simulink model "skipper_lqi_for_export"  (R2025b)
settings: Solver=FixedStepDiscrete  StartTime=0.0  StopTime=100  RelTol=1e-3
values from neighbouring files (symbols this model uses):
  A = [ ... (first row only)    [lqrMatrices.m]    (also in state_space.m)
  B = [ ... (first row only)    [lqrMatrices.m]    (also in state_space.m)
  C = diag(ones(1, 12))    [lqrMatrices.m]    (also in state_space.m = eye(12))
  D = zeros(size(B))    [lqrMatrices.m]    (also in state_space.m)
  d = [-rho 0 0]'    [derive_eom.m]    (also in lqrMatrices.m = [; state_space.m = [)
  K1 = Ki(:, 1:12)    [state_space.m]
  K2 = Ki(:, 13:end)    [state_space.m]
  qq = diag([1 1 1 0.001 0.001 0.001 1 1 1 0.001 0.001 0.001])    [state_space.m]
  Uff = -pinv(B)*d    [state_space.m]
undefined symbols (not defined in the file or in its folder): DiscIntNeverNeededParam, Discrete, Time
libraries: ctrlSharedLib x1
settings Model: Creator=nehir  LastModifiedBy=turbohirbo
settings OptimizationCC: DefaultParameterBehavior=Inlined  UseDivisionForNetSlopeComputation=on  GainParamInheritBuiltInType=on  UseFloatMulNetSlope=on  InlineInvariantSignals=on  ZeroExternalMemoryAtStartup=off  ZeroInternalMemoryAtStartup=off  EfficientFloat2IntCast=on  LifeSpan=1  OptimizeDataStoreBuffers=off  BusAssignmentInplaceUpdate=off
settings DebuggingCC: SFUnexpectedBacktrackingDiag=warning  SFNoUnconditionalDefaultTransitionDiag=warning
settings HardwareCC: ProdBitPerPointer=32.0  ProdBitPerSizeT=32.0  ProdBitPerPtrDiffT=32.0  ProdLargestAtomicInteger=Long  ProdLargestAtomicFloat=Double  ProdWordSize=32.0  ProdHWDeviceType=ARM Compatible->ARM Cortex-M
settings SFSimCC: MATLABDynamicMemAlloc=off
settings RTWCC: GenCodeOnly=on  GenerateReport=on  Toolchain=CMake  LaunchReport=on  TargetLang=C++
settings CodeAppCC: ForceParamTrailComments=on  EnableCustomComments=on
settings GRTTargetCC: MultiInstanceErrorCode=Warning  TargetLangStandard=C++17 (ISO)  CombineSignalStateStructs=on  MatFileLogging=off  CodeInterfacePackaging=C++ class  SupportVariableSizeSignals=on
settings SimscapeCC: SimscapeLogDecimation=1  SimscapeLogDataHistory=5000

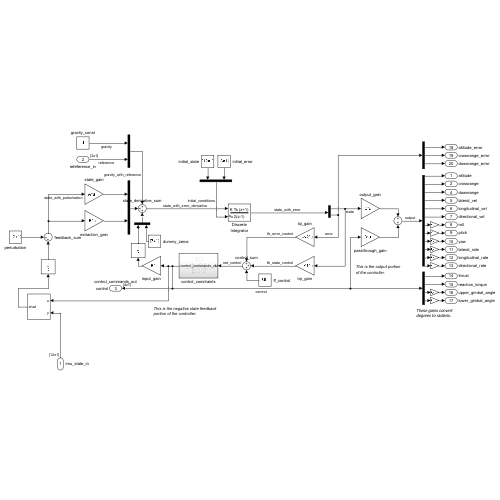
[thumbnail: Simulink's stored preview of the top-level diagram]
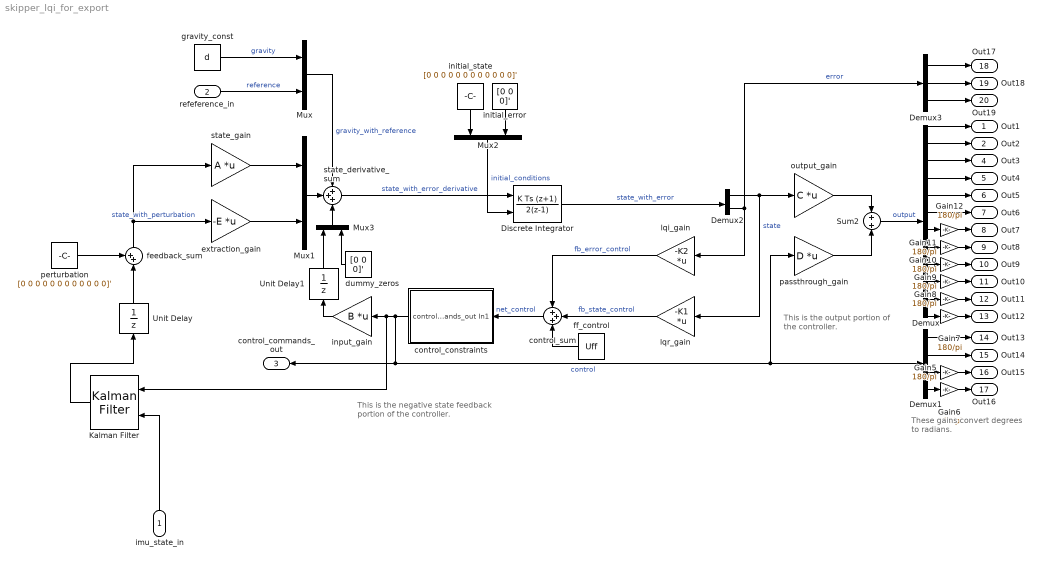
== system skipper_lqi_for_export ==
  note: This is the output portion
      | of the controller.
  note: This is the negative state feedback
      | portion of the controller.
  note: These gains convert
      | degrees to radians.
  imu_state_in : Inport  PortDimensions=[12 1]
  refeference_in : Inport  Port=2  PortDimensions=[3 1]
  Demux : Demux  Outputs=12
  Demux1 : Demux
  Demux2 : Demux  Outputs=[12 3]
  Demux3 : Demux  Outputs=3
  Discrete Integrator : DiscreteIntegrator  IntegratorMethod=Integration: Trapezoidal  InitialConditionSource=external  SampleTime=0.05  ICPrevOutput=DiscIntNeverNeededParam  ICPrevScaledInput=DiscIntNeverNeededParam
  Gain{5..12} (8 alike) : Gain  Gain=180/pi
  Kalman Filter : ctrlSharedLib/Kalman Filter  TimeDomain=Discrete-Time  UseCurrentEstimator=on  ModelSource=Individual A, B, C, D matrices  ModelSourceVariable=ss(0.95,1,1,0,1)  A=A  B=B  C=C  D=D  NumberOfStates=1  NumberOfInputs=1  NumberOfOutputs=1  InitialEstimateSource=Dialog  X0=0  P0=10  UseK=off  UseGH=off  NumberOfProcessNoiseInputs=1  G=1  TimeInvariantG=on  H=0  TimeInvariantH=on  Q=qq ./ 1  TimeInvariantQ=on  R=.01  TimeInvariantR=on  N=0  TimeInvariantN=on  AddInputPort=on  AddEnablePort=off  OutputEstimatedY=off  OutputP=off  Ts=-1
  Mux{,1..3} (4 alike) : Mux  Inputs=2
  Sum2 : Sum  Inputs=+|+
  Unit Delay : UnitDelay  SampleTime=0.05  HasFrameUpgradeWarning=on
  Unit Delay1 : UnitDelay  SampleTime=0.05  HasFrameUpgradeWarning=on
  control_constraints : Subsystem
  control_sum : Sum  Inputs=+++
  dummy_zeros : Constant  Value=[0 0 0]'  OutDataTypeStr=Inherit: Inherit via back propagation
  extraction_gain : Gain  Gain=-E  Multiplication=Matrix(K*u)
  feedback_sum : Sum  Inputs=++|
  ff_control : Constant  Value=Uff
  gravity_const : Constant  Value=d  OutDataTypeStr=double
  initial_error : Constant  Value=[0 0 0]'
  initial_state : Constant  Value=[0 0 0 0 0 0 0 0 0 0 0 0]'
  input_gain : Gain  Gain=B  Multiplication=Matrix(K*u)
  lqi_gain : Gain  Gain=-K2  Multiplication=Matrix(K*u)
  lqr_gain : Gain  Gain=-K1  Multiplication=Matrix(K*u)
  output_gain : Gain  Gain=C  Multiplication=Matrix(K*u)
  passthrough_gain : Gain  Gain=D  Multiplication=Matrix(K*u)
  perturbation : Constant  Value=[0 0 0 0 0 0 0 0 0 0 0 0]'
  state_derivative_sum : Sum  Inputs=+++
  state_gain : Gain  Gain=A  Multiplication=Matrix(K*u)
  Out1 : Outport  SignalName=altitude  Unit=ft
  Out2 : Outport  Port=2  SignalName=crossrange  Unit=ft
  control_commands_out : Outport  Port=3  SignalName=control  PortDimensions=[4 1]
  Out3 : Outport  Port=4  SignalName=downrange  Unit=ft
  Out4 : Outport  Port=5  SignalName=lateral_vel  Unit=ft/s
  Out5 : Outport  Port=6  SignalName=longitudinal_vel  Unit=ft/s
  Out6 : Outport  Port=7  SignalName=directional_vel  Unit=ft/s
  Out7 : Outport  Port=8  SignalName=roll  Unit=deg
  Out8 : Outport  Port=9  SignalName=pitch  Unit=deg
  Out9 : Outport  Port=10  SignalName=yaw  Unit=deg
  Out10 : Outport  Port=11  SignalName=lateral_rate  Unit=deg/s
  Out11 : Outport  Port=12  SignalName=longitudinal_rate  Unit=deg/s
  Out12 : Outport  Port=13  SignalName=directional_rate  Unit=deg/s
  Out13 : Outport  Port=14  SignalName=thrust  Unit=lbf
  Out14 : Outport  Port=15  SignalName=reaction_torque  Unit=lbf*ft
  Out15 : Outport  Port=16  SignalName=upper_gimbal_angle  Unit=deg
  Out16 : Outport  Port=17  SignalName=lower_gimbal_angle  Unit=deg
  Out17 : Outport  Port=18  SignalName=altitude_error  Unit=ft*s
  Out18 : Outport  Port=19  SignalName=crossrange_error  Unit=ft*s
  Out19 : Outport  Port=20  SignalName=downrange_error  Unit=ft*s
  wires:
  state_gain/1 -> Mux1/1
  input_gain/1 -> Unit Delay1/1
  state_derivative_sum/1 -> Discrete Integrator/1  "state_with_error_derivative"
  Discrete Integrator/1 -> Demux2/1  "state_with_error"
  output_gain/1 -> Sum2/1
  passthrough_gain/1 -> Sum2/2
  ff_control/1 -> control_sum/3
  lqr_gain/1 -> control_sum/2  "fb_state_control"
  control_sum/1 -> control_constraints/1(In1)  "net_control"
  initial_state/1 -> Mux2/1
  Sum2/1 -> Demux/1  "output"
  Demux/1 -> Out1/1
  Demux/2 -> Out2/1
  Demux/3 -> Out3/1
  Demux/4 -> Out4/1
  Demux/5 -> Out5/1
  Demux/6 -> Out6/1
  Demux1/1 -> Out13/1
  Demux1/2 -> Out14/1
  Demux1/3 -> Gain5/1
  Gain5/1 -> Out15/1
  Gain6/1 -> Out16/1
  Demux1/4 -> Gain6/1
  Demux/12 -> Gain7/1
  Gain7/1 -> Out12/1
  Demux/11 -> Gain8/1
  Demux/9 -> Gain10/1
  Demux/7 -> Gain12/1
  Demux/8 -> Gain11/1
  Demux/10 -> Gain9/1
  Gain12/1 -> Out7/1
  Gain11/1 -> Out8/1
  Gain10/1 -> Out9/1
  Gain9/1 -> Out10/1
  Gain8/1 -> Out11/1
  gravity_const/1 -> Mux/1  "gravity"
  refeference_in/1 -> Mux/2  "reference"
  extraction_gain/1 -> Mux1/2
  Mux1/1 -> state_derivative_sum/2
  Mux/1 -> state_derivative_sum/1  "gravity_with_reference"
  Demux2/1 -> lqr_gain/1, output_gain/1  "state"
  Demux2/2 -> Demux3/1, lqi_gain/1  "error"
  lqi_gain/1 -> control_sum/1  "fb_error_control"
  initial_error/1 -> Mux2/2
  Mux2/1 -> Discrete Integrator/2  "initial_conditions"
  Mux3/1 -> state_derivative_sum/3
  dummy_zeros/1 -> Mux3/2
  Demux3/3 -> Out19/1
  Demux3/2 -> Out18/1
  Demux3/1 -> Out17/1
  feedback_sum/1 -> state_gain/1, extraction_gain/1  "state_with_perturbation"
  perturbation/1 -> feedback_sum/1
  control_constraints/1(control_commands_out) -> control_commands_out/1, Demux1/1, passthrough_gain/1, Kalman Filter/1, input_gain/1  "control"
  Unit Delay/1 -> feedback_sum/2
  Unit Delay1/1 -> Mux3/1
  imu_state_in/1 -> Kalman Filter/2
  Kalman Filter/1 -> Unit Delay/1

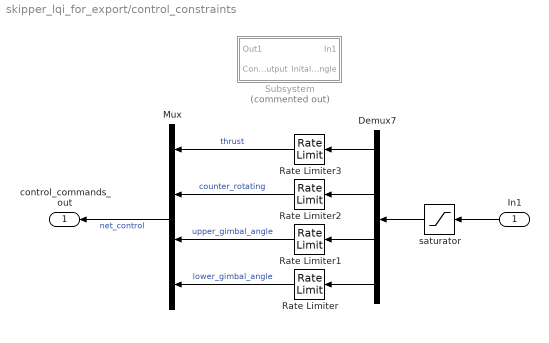
== system skipper_lqi_for_export/control_constraints ==
  In1 : Inport
  Demux7 : Demux  Outputs=[1 1 1 1]
  Mux : Mux
  Rate Limiter : RateLimiter  RisingSlewLimit=inf  FallingSlewLimit=-inf  SampleTimeMode=inherited  InitialCondition=1.7
  Rate Limiter1 : RateLimiter  RisingSlewLimit=inf  FallingSlewLimit=-inf  SampleTimeMode=inherited  InitialCondition=1.7
  Rate Limiter2 : RateLimiter  RisingSlewLimit=inf  FallingSlewLimit=-inf  SampleTimeMode=inherited  InitialCondition=1.7
  Rate Limiter3 : RateLimiter  RisingSlewLimit=inf  FallingSlewLimit=-inf  SampleTimeMode=inherited
  Subsystem : Subsystem  Commented=on
  saturator : Saturate  UpperLimit=[3.5 1 pi/22 pi/22]'  LowerLimit=[0 -1 -pi/22 -pi/22]'
  control_commands_out : Outport
  wires:
  Mux/1 -> control_commands_out/1  "net_control"
  In1/1 -> saturator/1
  Rate Limiter3/1 -> Mux/1  "thrust"
  Rate Limiter/1 -> Mux/4  "lower_gimbal_angle"
  Rate Limiter1/1 -> Mux/3  "upper_gimbal_angle"
  Rate Limiter2/1 -> Mux/2  "counter_rotating"
  Demux7/1 -> Rate Limiter3/1
  Demux7/2 -> Rate Limiter2/1
  Demux7/3 -> Rate Limiter1/1
  Demux7/4 -> Rate Limiter/1
  saturator/1 -> Demux7/1

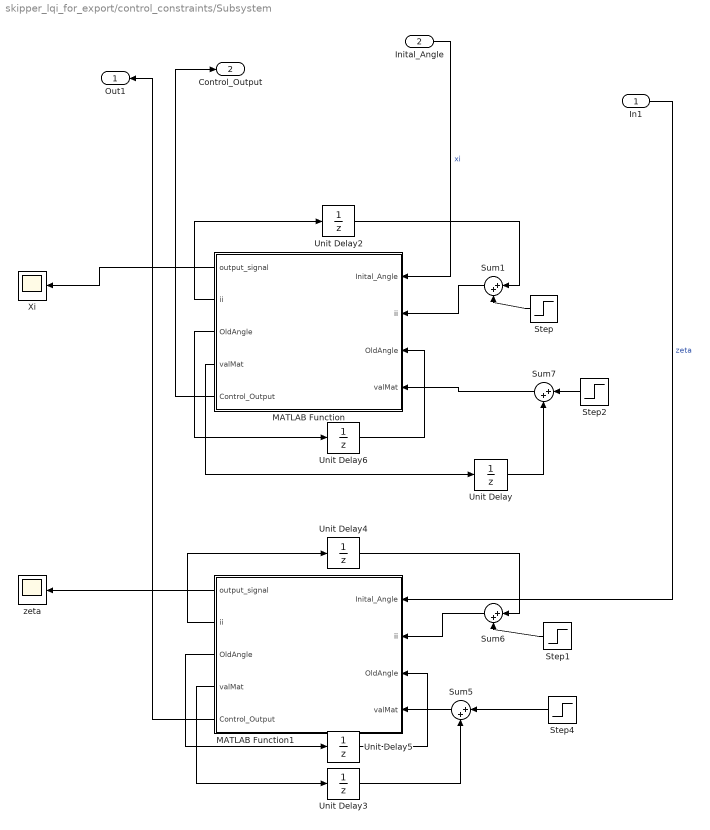
== system skipper_lqi_for_export/control_constraints/Subsystem ==
  In1 : Inport
  Inital_Angle : Inport  Port=2
  MATLAB Function : MATLAB Function  TreatAsAtomicUnit=on
  MATLAB Function1 : MATLAB Function  TreatAsAtomicUnit=on
  Step : Step  Before=1  After=0  SampleTime=0
  Step1 : Step  Before=1  After=0  SampleTime=0
  Step2 : Step  Time=0  After=[0 0 0 0 0 0 0 0 0 0]  SampleTime=0  VectorParams1D=off
  Step4 : Step  Time=0  After=[0 0 0 0 0 0 0 0 0 0]  SampleTime=0  VectorParams1D=off
  Sum{1,5..7} (4 alike) : Sum  Inputs=|++
  Unit Delay{,2..6} (6 alike) : UnitDelay  SampleTime=0.01  HasFrameUpgradeWarning=on
  Xi : Scope
      settings: ActiveDisplayYMinimum=1480.36505  ActiveDisplayYMaximum=1519.63495
  zeta : Scope
      settings: ActiveDisplayYMinimum=1497.81834  ActiveDisplayYMaximum=1502.18166  DataLoggingVariableName=ScopeData2
  Out1 : Outport
  Control_Output : Outport  Port=2
  wires:
  Unit Delay3/1 -> Sum5/2
  MATLAB Function/4(valMat) -> Unit Delay/1
  Step2/1 -> Sum7/1
  Step1/1 -> Sum6/2
  MATLAB Function1/5(Control_Output) -> Out1/1
  MATLAB Function/2(ii) -> Unit Delay2/1
  MATLAB Function1/2(ii) -> Unit Delay4/1
  In1/1 -> MATLAB Function1/1(Inital_Angle)  "zeta"
  Sum5/1 -> MATLAB Function1/4("valMat ")
  Unit Delay/1 -> Sum7/2
  Unit Delay5/1 -> MATLAB Function1/3("OldAngle ")
  Sum6/1 -> MATLAB Function1/2("ii ")
  Inital_Angle/1 -> MATLAB Function/1(Inital_Angle)  "xi"
  Unit Delay2/1 -> Sum1/1
  MATLAB Function1/4(valMat) -> Unit Delay3/1
  MATLAB Function/5(Control_Output) -> Control_Output/1
  MATLAB Function1/1(output_signal) -> zeta/1
  Sum7/1 -> MATLAB Function/4("valMat ")
  Step4/1 -> Sum5/1
  Step/1 -> Sum1/2
  Unit Delay6/1 -> MATLAB Function/3("OldAngle ")
  MATLAB Function/3(OldAngle) -> Unit Delay6/1
  Unit Delay4/1 -> Sum6/1
  MATLAB Function1/3(OldAngle) -> Unit Delay5/1
  MATLAB Function/1(output_signal) -> Xi/1
  Sum1/1 -> MATLAB Function/2("ii ")

== matlab function skipper_lqi_for_export/control_constraints/Subsystem/MATLAB Function ==
  data: Inital_Angle input; output_signal output; ii input; OldAngle input; valMat input; ii output; OldAngle output; valMat output; Control_Output output
function [output_signal, ii, OldAngle, valMat, Control_Output] = FRL_Gimbal(Inital_Angle, ii, OldAngle, valMat)

%Initilizing Variables

% ii = 1, OldAv =0;
%valMat = [0 0 0 0 0 0 0 0 0 0];
% IAV = input angular velocity
maxAngle = 10;
minAngle = -10;

if Inital_Angle > maxAngle
    Inital_Angle = maxAngle;
elseif Inital_Angle <minAngle
    Inital_Angle = minAngle;
end 


%maxAngleError = 3;
MaxPWMSignal = 2500;
Min_PWM_Singal = 500;

% Rotating IAV matrix
valMat(ii) = Inital_Angle;
ii = ii+1;

%looping ii if it goes over 10
if ii >= 10
    ii =1;
end

%finding adverage value of matrix
ValMatAdv = 0;
for jj = 1:1:10
ValMatAdv = ValMatAdv + valMat(jj);
end
ValMatAdv = ValMatAdv / 10;
NewAngle = ValMatAdv;

%If the adverage value is near zero clear to remove occilation
%discontiunity
if (abs(NewAngle - OldAngle) < .001)
    valMat = [0 0 0 0 0 0 0 0 0 0];
end


%if angle is outside range set to max angle
if NewAngle > maxAngle
    NewAngle = maxAngle;
elseif NewAngle < minAngle
    NewAngle = minAngle;
end

%calculate final signal
output_signal = ((MaxPWMSignal - Min_PWM_Singal) * (NewAngle/(maxAngle-minAngle))) +( Min_PWM_Singal + (MaxPWMSignal -Min_PWM_Singal)/2);

OldAngle = NewAngle;
Control_Output = NewAngle;
end

== matlab function skipper_lqi_for_export/control_constraints/Subsystem/MATLAB Function1 ==
  data: Inital_Angle input; output_signal output; ii input; OldAngle input; valMat input; ii output; OldAngle output; valMat output; Control_Output output
function [output_signal, ii, OldAngle, valMat, Control_Output] = FRL_Gimbal(Inital_Angle, ii, OldAngle, valMat)

%Initilizing Variables

% ii = 1, OldAv =0;
%valMat = [0 0 0 0 0 0 0 0 0 0];
% IAV = input angular velocity
maxAngle = 10;
minAngle = -10;

if Inital_Angle > maxAngle
    Inital_Angle = maxAngle;
elseif Inital_Angle <minAngle
    Inital_Angle = minAngle;
end


%maxAngleError = 3;
MaxPWMSignal = 2500;
Min_PWM_Singal = 500;

% Rotating IAV matrix
valMat(ii) = Inital_Angle;
ii = ii+1;

%looping ii if it goes over 10
if ii >= 10
    ii =1;
end

%finding adverage value of matrix
ValMatAdv = 0;
for jj = 1:1:10
ValMatAdv = ValMatAdv + valMat(jj);
end
ValMatAdv = ValMatAdv / 10;
NewAngle = ValMatAdv;

%If the adverage value is near zero clear to remove occilation
%discontiunity
if (abs(NewAngle - OldAngle) < .001)
    valMat = [0 0 0 0 0 0 0 0 0 0];
end


%if angle is outside range set to max angle
if NewAngle > maxAngle
    NewAngle = maxAngle;
elseif NewAngle < minAngle
    NewAngle = minAngle;
end

%calculate final signal
output_signal = ((MaxPWMSignal - Min_PWM_Singal) * (NewAngle/(maxAngle-minAngle))) +( Min_PWM_Singal + (MaxPWMSignal -Min_PWM_Singal)/2);

OldAngle = NewAngle;
Control_Output = NewAngle;
end
